simulink model "adaptive"  (R2019a)
settings: Solver=VariableStepAuto  StartTime=0.0  StopTime=50  RelTol=1e-3
libraries: simulink x1
settings Model: Creator=24249  LastModifiedBy=24249

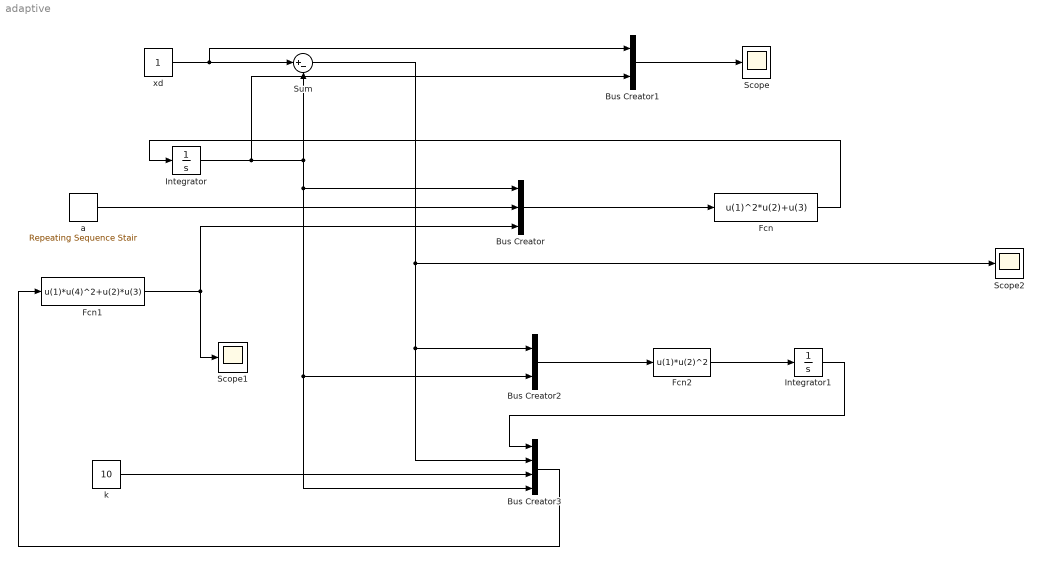
== system adaptive ==
  Bus Creator : BusCreator  Inputs=3
  Bus Creator1 : BusCreator  Inputs=2
  Bus Creator2 : BusCreator  Inputs=2
  Bus Creator3 : BusCreator  Inputs=4
  Fcn : Fcn  Expr=u(1)^2*u(2)+u(3)
  Fcn1 : Fcn  Expr=u(1)*u(4)^2+u(2)*u(3)
  Fcn2 : Fcn  Expr=u(1)*u(2)^2
  Integrator : Integrator
  Integrator1 : Integrator
  Scope : Scope
  Scope1 : Scope
  Scope2 : Scope
  Sum : Sum  Inputs=|+-
  a : simulink/Sources/Repeating Sequence Stair  OutValues=[1 2].'  tsamp=-1  OutMin=[]  OutMax=[]  OutDataTypeStr=double  OutputDataTypeScalingMode=double  OutDataType=fixdt(0,8)  ConRadixGroup=Best Precision: Vector-wise  OutScaling=2^-12
  k : Constant  Value=10
  xd : Constant
  wires:
  xd/1 -> Bus Creator1/1, Sum/1
  Integrator/1 -> Bus Creator1/2, Bus Creator3/4, Bus Creator2/2, Bus Creator/1, Sum/2
  Fcn/1 -> Integrator/1
  Bus Creator/1 -> Fcn/1
  Sum/1 -> Scope2/1, Bus Creator2/1, Bus Creator3/2
  Bus Creator2/1 -> Fcn2/1
  Fcn2/1 -> Integrator1/1
  Integrator1/1 -> Bus Creator3/1
  k/1 -> Bus Creator3/3
  a/1 -> Bus Creator/2
  Fcn1/1 -> Scope1/1, Bus Creator/3
  Bus Creator3/1 -> Fcn1/1
  Bus Creator1/1 -> Scope/1
